simulink model "vector_field"  (R2015a)
settings: Solver=ode45  StartTime=0.0  StopTime=100.0  RelTol=1e-3
values from neighbouring files (symbols this model uses):
  a = (y_end-y_int)/(x_end-x_int)    [vector_st.m]    (also in vf.m = 0.5)
  alpha = 1.65    [vector_st.m]    (also in vf.m)
  ang = atan2(y_end-y_int,x_end-x_int)    [vector_st.m]    (also in vf.m = atan2(150,300))
  b = y_end-x_end*a    [vector_st.m]    (also in vf.m = 0)
  chi_inf = pi/2    (= 1.57079632679)    [vector_st.m]    (also in vf.m)
  course_int = 0    [vector_st.m]    (also in vf.m)
  epsi = 0.1    [vector_st.m]    (also in vf.m)
  i = -1    [vector_st.m]    (also in vf.m)
  k = mag-r    [lyapunov_vf.m]    (also in vector_st.m = 0.02; vf.m = 0.02)
  kk = pi/2    (= 1.57079632679)    [vector_st.m]    (also in vf.m = har(j))
  phiw = 230/180*pi    (= 4.01425727959)    [vector_st.m]    (also in vf.m)
  Va = 10    [vector_st.m]    (also in vf.m = 13)
  w = 0    [vector_st.m]    (also in vf.m)
  x_int = -100    [lsl.m]    (also in lyapunov_vf.m; lyapunov_vf_3d.m = 20; rsl.m = -300; vf.m = 0)
  y_int = 10    [lsl.m]    (also in lyapunov_vf.m = -200; lyapunov_vf_3d.m = 20; rsl.m = 0; vf.m = -50)
undefined symbols (not defined in the file or in its folder): x_end
libraries: simulink x1
settings Model: Creator=KVV  LastModifiedBy=KVV

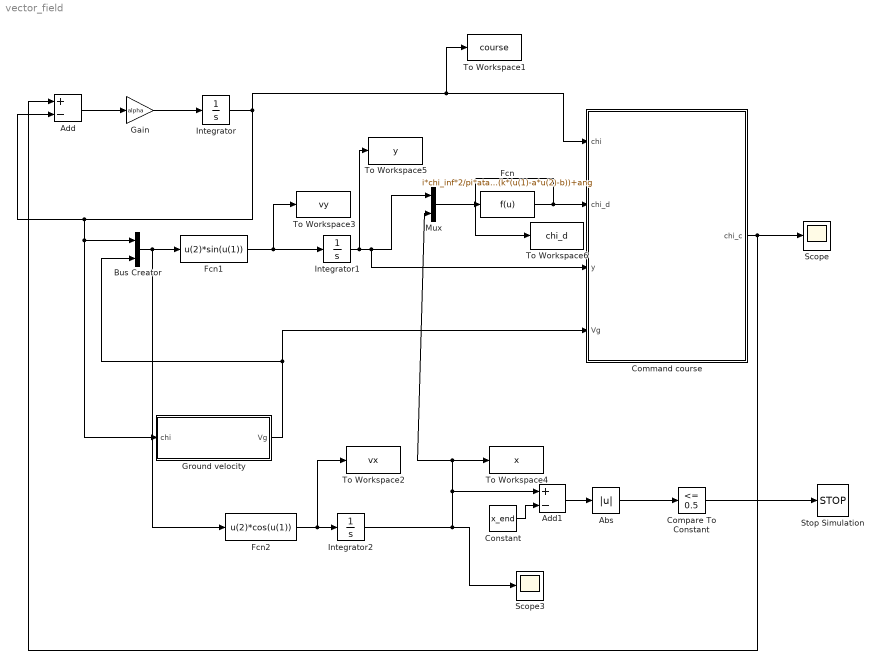
== system vector_field ==
  Abs : Abs
  Add : Sum  Inputs=+-
  Add1 : Sum  Inputs=+-
  Bus Creator : BusCreator  Inputs=2
  Command course : Subsystem
  Compare To Constant : simulink/Logic and Bit Operations/Compare To Constant  relop=<=  const=0.5  OutDataTypeStr=boolean
  Constant : Constant  Value=x_end
  Fcn : Fcn  Expr=i*chi_inf*2/pi*atan(k*(u(1)-a*u(2)-b))+ang
  Fcn1 : Fcn  Expr=u(2)*sin(u(1))
  Fcn2 : Fcn  Expr=u(2)*cos(u(1))
  Gain : Gain  Gain=alpha
  Ground velocity : Subsystem
  Integrator : Integrator  InitialCondition=course_int
  Integrator1 : Integrator  InitialCondition=y_int
  Integrator2 : Integrator  InitialCondition=x_int
  Mux : Mux  Inputs=2
  Scope : Scope
  Scope3 : Scope
      settings: YMin=-945.33421  YMax=140.26448  SaveName=ScopeData3
  Stop Simulation : Stop
  To Workspace1 : ToWorkspace  VariableName=course  SaveFormat=Timeseries  SampleTime=-1
  To Workspace2 : ToWorkspace  VariableName=vx  SaveFormat=Timeseries  SampleTime=-1
  To Workspace3 : ToWorkspace  VariableName=vy  SaveFormat=Timeseries  SampleTime=-1
  To Workspace4 : ToWorkspace  VariableName=x  SaveFormat=Timeseries  SampleTime=-1
  To Workspace5 : ToWorkspace  VariableName=y  SaveFormat=Timeseries  SampleTime=-1
  To Workspace6 : ToWorkspace  VariableName=chi_d  SaveFormat=Timeseries  SampleTime=-1
  wires:
  Add/1 -> Gain/1
  Gain/1 -> Integrator/1
  Integrator/1 -> Add/2, Bus Creator/1, Ground velocity/1(chi), To Workspace1/1, Command course/1(chi)
  Ground velocity/1(Vg) -> Command course/4(Vg), Bus Creator/2
  Fcn1/1 -> Integrator1/1, To Workspace3/1
  Integrator1/1 -> To Workspace5/1, Command course/3(y), Mux/1
  Fcn2/1 -> To Workspace2/1, Integrator2/1
  Mux/1 -> Fcn/1
  Fcn/1 -> To Workspace6/1, Command course/2(chi_d)
  Command course/1(chi_c) -> Scope/1, Add/1
  Bus Creator/1 -> Fcn2/1, Fcn1/1
  Integrator2/1 -> Add1/1, Mux/2, To Workspace4/1, Scope3/1
  Constant/1 -> Add1/2
  Add1/1 -> Abs/1
  Abs/1 -> Compare To Constant/1
  Compare To Constant/1 -> Stop Simulation/1

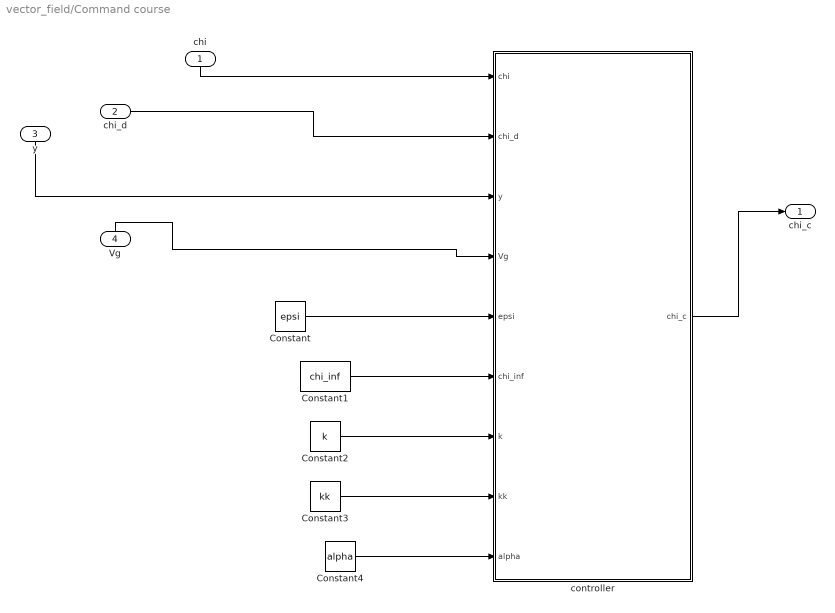
== system vector_field/Command course ==
  chi : Inport
  chi_d : Inport  Port=2
  y : Inport  Port=3
  Vg : Inport  Port=4
  Constant : Constant  Value=epsi
  Constant1 : Constant  Value=chi_inf
  Constant2 : Constant  Value=k
  Constant3 : Constant  Value=kk
  Constant4 : Constant  Value=alpha
  controller : MATLAB Function  TreatAsAtomicUnit=on
  chi_c : Outport
  wires:
  Constant4/1 -> controller/9(alpha)
  y/1 -> controller/3(y)
  Constant3/1 -> controller/8(kk)
  Constant2/1 -> controller/7(k)
  Constant/1 -> controller/5(epsi)
  Constant1/1 -> controller/6(chi_inf)
  Vg/1 -> controller/4(Vg)
  chi/1 -> controller/1(chi)
  controller/1(chi_c) -> chi_c/1
  chi_d/1 -> controller/2(chi_d)

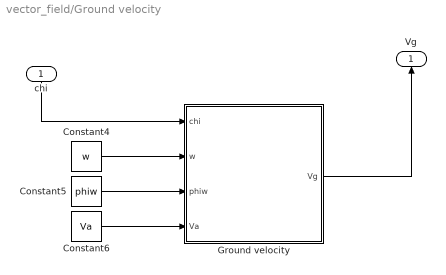
== system vector_field/Ground velocity ==
  chi : Inport
  Constant4 : Constant  Value=w
  Constant5 : Constant  Value=phiw
  Constant6 : Constant  Value=Va
  Ground velocity : MATLAB Function  TreatAsAtomicUnit=on
  Vg : Outport
  wires:
  Constant4/1 -> Ground velocity/2(w)
  Constant5/1 -> Ground velocity/3(phiw)
  Constant6/1 -> Ground velocity/4(Va)
  chi/1 -> Ground velocity/1(chi)
  Ground velocity/1(Vg) -> Vg/1

== matlab function vector_field/Ground velocity/Ground velocity ==
  data: chi input; Vg output; w input; phiw input; Va input
function Vg = GroundVelocity(chi,w,phiw,Va)
%generate the ground velocity based on course angle
Vg=w*cos(chi-phiw)+sqrt(Va^2-w^2*(sin(chi-phiw))^2);
end

== matlab function vector_field/Command course/controller ==
  data: chi input; chi_d input; y input; Vg input; chi_c output; epsi input; chi_inf input; k input; kk input; alpha input
function chi_c = CommandCourse(chi,chi_d,y,Vg,epsi,chi_inf,k,kk,alpha)
%generate command course angle chi_c
sat=(chi-chi_d)/epsi;
if abs(sat)<=1
    rho=sat;
else
    rho=sign(sat);
end
chi_c=chi-chi_inf*2/pi/alpha*k/(1+(k*y)^2)*Vg*sin(chi)-kk/alpha*rho;


end
